simulink model "StewartPlatform"  (R2024a)
settings: Solver=ode8  StartTime=0.0  StopTime=inf  FixedStep=0.02  RelTol=1e-3  EnableMultiTasking=on
undefined symbols (not defined in the file or in its folder): Camera, Standard_Devices
libraries: pycoexlib x1, visionsinks x1, sldrtlib x1
settings Model: SimulationMode=external  ExtModeTrigDuration=2  Creator=Acrome  LastModifiedBy=burli
settings SolverCC: AlgebraicLoopSolver=TrustRegion
settings DataIOCC: ReturnWorkspaceOutputs=off
settings OptimizationCC: PassReuseOutputArgsAs=Individual arguments  MaxStackSize=64  EfficientTunableParamExpr=on
settings DebuggingCC: ParameterTunabilityLossMsg=error  UnconnectedInputMsg=warning  UnconnectedOutputMsg=warning  UnconnectedLineMsg=warning  ArithmeticOperatorsInVariantConditions=warning
settings HardwareCC: ProdBitPerInt=16  ProdBitPerPointer=16  ProdBitPerSizeT=16  ProdBitPerPtrDiffT=16  ProdLargestAtomicFloat=None  ProdWordSize=8  ProdHWDeviceType=Atmel->AVR
settings ModelReferenceCC: EnableRefExpFcnMdlSchedulingChecks=on
settings SFSimCC: SimUseLocalCustomCode=off  MATLABDynamicMemAlloc=off  CustomCodeUndefinedFunction=UseInterfaceOnly
settings RTWCC: Description=Embedded Coder  SystemTargetFile=ert.tlc  HardwareBoard=Arduino Mega 2560  TemplateMakefile=ert_default_tmf  GenerateReport=on  RTWUseLocalCustomCode=off  Toolchain=Arduino AVR  BuildConfiguration=Faster Runs  IncludeHyperlinkInReport=on  LaunchReport=on  GenerateTraceInfo=on  GenerateTraceReport=on  GenerateTraceReportSl=on  GenerateTraceReportSf=on  GenerateTraceReportEml=on  GPUComputeCapability=3.5
settings CodeAppCC: ForceParamTrailComments=on  IgnoreCustomStorageClasses=off  OperatorAnnotations=on  SimulinkDataObjDesc=on  SFDataObjDesc=on  InsertBlockDesc=on
settings ERTTargetCC: SupportContinuousTime=on  SupportVariableSizeSignals=on  ExtMode=on  ExtModeTransport=3  ExtModeStaticAlloc=on  ExtModeMexFile=ext_xcp  ExtModeMexArgs='127.0.0.1' 0 17725  ExtModeIntrfLevel=Level2 - Open

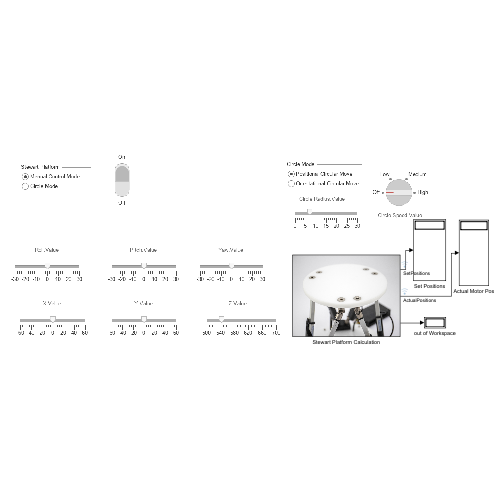
[thumbnail: Simulink's stored preview of the top-level diagram]
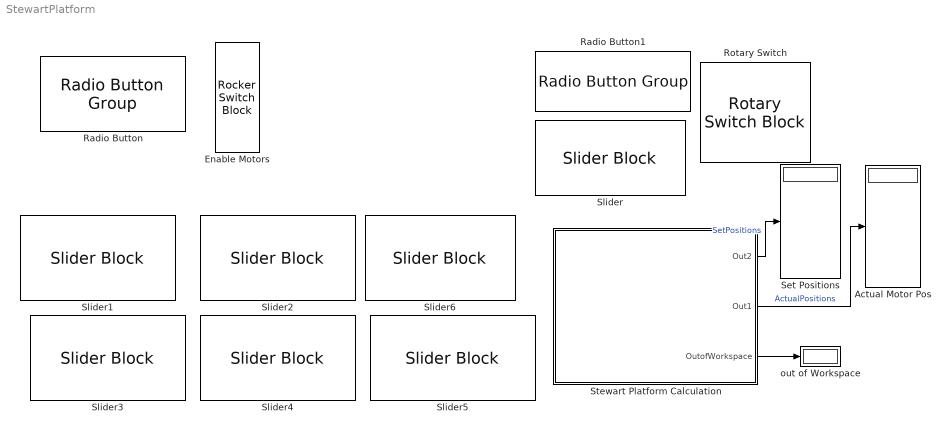
== system StewartPlatform ==
  Actual Motor Pos : Display
  Enable Motors : RockerSwitchBlock  LabelPosition=Hide
      settings: Values={{'Off', 'On'}, [0 1]}
  Radio Button : RadioButtonGroup  LabelPosition=Hide  SelectedLabel=Manual Control Mode  ButtonGroupName=Stewart Platform
      settings: Values={{'Manual Control Mode', 'Circle Mode'}, [0 1]}
  Radio Button1 : RadioButtonGroup  LabelPosition=Hide  SelectedLabel=Positional Circular Move  ButtonGroupName=Circle Mode
      settings: Values={{'Positional Circular Move', 'Orientational Circular Move'}, [0 1]}
  Rotary Switch : RotarySwitchBlock  LabelPosition=Bottom
      settings: Values={{'Off', 'Low', 'Medium', 'High'}, [0 2 3 4]}
  Set Positions : Display
  Slider : SliderBlock  ScaleMax=30
  Slider1 : SliderBlock  ScaleMin=-30  ScaleMax=30  TickInterval=10
  Slider2 : SliderBlock  ScaleMin=-30  ScaleMax=30  TickInterval=10
  Slider3 : SliderBlock  ScaleMin=-60  ScaleMax=60  TickInterval=20
  Slider4 : SliderBlock  ScaleMin=-60  ScaleMax=60  TickInterval=20
  Slider5 : SliderBlock  ScaleMin=500  ScaleMax=700
  Slider6 : SliderBlock  ScaleMin=-30  ScaleMax=30  TickInterval=10
  Stewart Platform Calculation : Subsystem
      mask Display: image('IMG_7112_1.jpg');
  out of Workspace : Display
  wires:
  Stewart Platform Calculation/2(Out1) -> Actual Motor Pos/1  "ActualPositions"
  Stewart Platform Calculation/1(Out2) -> Set Positions/1  "SetPositions"
  Stewart Platform Calculation/3(OutofWorkspace) -> out of Workspace/1

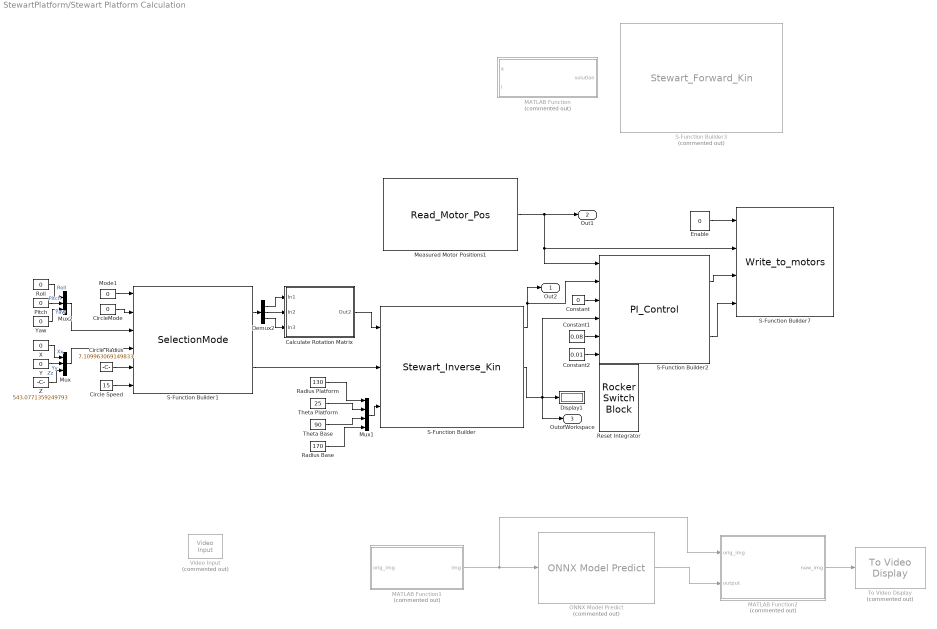
== system StewartPlatform/Stewart Platform Calculation ==
  " X" : Constant  Value=0
  Calculate Rotation Matrix : Subsystem
  Circle Radius : Constant  Value=7.109963069149833
  Circle Speed : Constant  Value=15
  CircleMode : Constant  Value=0  SampleTime=-1
  Constant : Constant  Value=0
  Constant1 : Constant  Value=0.08
  Constant2 : Constant  Value=0.01
  Demux2 : Demux  Outputs=3
  Display1 : Display
  Enable : Constant  Value=0
  MATLAB Function : MATLAB Function  Commented=on  TreatAsAtomicUnit=on
  MATLAB Function1 : MATLAB Function  Commented=on  TreatAsAtomicUnit=on
  MATLAB Function2 : MATLAB Function  Commented=on  TreatAsAtomicUnit=on
  Measured Motor Positions1 : S-Function  InitFcn=try, set_param(gcb,'FunctionName','Read_Motor_Pos'), end  FunctionName=Read_Motor_Pos  SFunctionModules=Read_Motor_Pos_wrapper.c  SFunctionDeploymentMode=off  EnableBusSupport=off  mask(S-Function Builder){}
      mask help: Simulink:masks:SFunctionBuilder_MD
      mask init:
      | val = [[.9  0.75 0.75 1 1 .9 .9 1]',[1 1 0.75 0.75 .9 .9 1 .9]'];try , sys = get_param(gcb,'SfunBuilderFcnName');if isempty(sys), sys = get_param(gcb,'FunctionName'); end,catch, sys = get_param(gcb,'FunctionName'); end
      settings: CopyFcn=set_param(gcbh,'LinkStatus','none')  PreSaveFcn=try, set_param(gcb,'FunctionName','Read_Motor_Pos'), end  OpenFcn=sfunctionwizard(gcbh)
      mask Display:
      | plot(val(:,1),val(:,2))
      | disp(sys)
      | port_label('output',1,'Mot_Pos')
  Mode1 : Constant  Value=0  SampleTime=-1
  Mux : Mux  Inputs=3
  Mux1 : Mux
  Mux2 : Mux  Inputs=3
  ONNX Model Predict : pycoexlib/ONNX Model Predict  Commented=on  ModelFile=C:\StewartProMatlab\SPro_Matlab_Mosfet v1_0_1\onnx_model_14.onnx  ExecutionProviders=CUDAExecutionProvider, CPUExecutionProvider  InputTable={ 'In1', 'float32', '[4 3 1 2]', 'inherit' }  OutputTable={ 'Out1', '', '' }  SampleTime=-1  InputDatatypes=float32  InputNumDims=inherit  InputPermutations=[4 3 1 2]  OutputPermutations=[]  PythonCoexecutionBlockType=ONNXModelBlock  VariableOutputMaxSizes=[]
  Pitch : Constant  Value=0  SampleTime=-1
  Radius Base : Constant  Value=170
  Radius Platform : Constant  Value=130
  Reset Integrator : RockerSwitchBlock  LabelPosition=Hide
      settings: Values={{'Off', 'On'}, [0 1]}
  Roll : Constant  Value=0  SampleTime=-1
  S-Function Builder : S-Function  InitFcn=try, set_param(gcb,'FunctionName','Stewart_Inverse_Kin'), end  FunctionName=Stewart_Inverse_Kin  SFunctionModules=Stewart_Inverse_Kin_wrapper  SFunctionDeploymentMode=off  EnableBusSupport=off  mask(S-Function Builder){}
      mask help: Simulink:masks:SFunctionBuilder_MD
      mask init: same as StewartPlatform/Stewart Platform Calculation/Measured Motor Positions1
      settings: CopyFcn=set_param(gcbh,'LinkStatus','none')  PreSaveFcn=try, set_param(gcb,'FunctionName','Stewart_Inverse_Kin'), end  OpenFcn=sfunctionwizard(gcbh)
      mask Display: plot(val(:,1),val(:,2)),disp(sys), port_label('input',1,'rotationmatrix'), port_label('input',2,'platform_pos'), port_label('input',3,'platform_parameters'), port_label('output',1,'Setpoints'), port_label('output',2,'outofWorkspace'), port_label('output',3,'y0')
  S-Function Builder1 : S-Function  InitFcn=try, set_param(gcb,'FunctionName','SelectionMode'), end  FunctionName=SelectionMode  SFunctionModules=SelectionMode_wrapper  SFunctionDeploymentMode=off  EnableBusSupport=off  mask(S-Function Builder){}
      mask help: Simulink:masks:SFunctionBuilder_MD
      mask init: same as StewartPlatform/Stewart Platform Calculation/Measured Motor Positions1
      settings: CopyFcn=set_param(gcbh,'LinkStatus','none')  PreSaveFcn=try, set_param(gcb,'FunctionName','SelectionMode'), end  OpenFcn=sfunctionwizard(gcbh)
      mask Display:
      | plot(val(:,1),val(:,2))
      | disp(sys)
      | port_label('input',1,'Mode')
      | port_label('input',2,'CircleMode')
      | port_label('input',3,'orientation_in')
      | port_label('input',4,'position_in')
      | port_label('input',5,'Radius')
      | port_label('input',6,'Speed')
      | port_label('output',1,'orientation_out')
      | port_label('output',2,'position_out')
  S-Function Builder2 : S-Function  InitFcn=try, set_param(gcb,'FunctionName','PI_Control'), end  FunctionName=PI_Control  SFunctionModules=PI_Control_wrapper  SFunctionDeploymentMode=off  EnableBusSupport=off  mask(S-Function Builder){}
      mask help: Simulink:masks:SFunctionBuilder_MD
      mask init: same as StewartPlatform/Stewart Platform Calculation/Measured Motor Positions1
      settings: CopyFcn=set_param(gcbh,'LinkStatus','none')  PreSaveFcn=try, set_param(gcb,'FunctionName','PI_Control'), end  OpenFcn=sfunctionwizard(gcbh)
      mask Display: plot(val(:,1),val(:,2)),disp(sys), port_label('input',1,'ActualPos'), port_label('input',2,'SetPos'), port_label('input',3,'ResetIntegrator'), port_label('input',4,'inWorkSpace'), port_label('input',5,'P'), port_label('input',6,'I'), port_label('output',1,'PWMOut'), port_label('output',2,'Directions')
  S-Function Builder3 : S-Function  Commented=on  FunctionName=Stewart_Forward_Kin  SFunctionModules=Stewart_Forward_Kin_wrapper.c  SFunctionDeploymentMode=off  EnableBusSupport=off  mask(S-Function Builder){}
      mask help: Simulink:masks:SFunctionBuilder_MD
      mask init: same as StewartPlatform/Stewart Platform Calculation/Measured Motor Positions1
      settings: CopyFcn=set_param(gcbh,'LinkStatus','none')  OpenFcn=sfunctionwizard(gcbh)
      mask Display:
      | plot(val(:,1),val(:,2))
      | disp(sys)
      | port_label('input',1,'actual_lengths')
      | port_label('input',2,'platform_parameters')
      | port_label('output',1,'actual_pos')
  S-Function Builder7 : S-Function  InitFcn=try, set_param(gcb,'FunctionName','Write_to_motors'), end  FunctionName=Write_to_motors  SFunctionModules=Write_to_motors_wrapper  SFunctionDeploymentMode=off  EnableBusSupport=off  mask(S-Function Builder){}
      mask help: Simulink:masks:SFunctionBuilder_MD
      mask init: same as StewartPlatform/Stewart Platform Calculation/Measured Motor Positions1
      settings: CopyFcn=set_param(gcbh,'LinkStatus','none')  PreSaveFcn=try, set_param(gcb,'FunctionName','Write_to_motors'), end  OpenFcn=sfunctionwizard(gcbh)
      mask Display: plot(val(:,1),val(:,2)),disp(sys),port_label('input',1,'EnabledMotors'),port_label('input',2,'MotorPos'),port_label('input',3,'PWMin'),port_label('input',4,'Direction')
  Theta Base : Constant  Value=90
  Theta Platform : Constant  Value=25
  To Video Display : visionsinks/To Video Display  Commented=on  windowSizeMode=Normal  openAtMdlStart=on  fullScreen=off  videoWindowX=536805376  videoWindowY=536805376  saveWindowSize=off  videoWindowWidth=2147483647  videoWindowHeight=2147483647  inputColorFormat=RGB  inputType=Obsolete  imagePorts=One multidimensional signal  OutputDevice=On-screen video monitor  dataOrg=Column-major  isWindowOpen=off
  Video Input : sldrtlib/Video Input  Commented=on  SampleTime=0.1  MaxMissedTicks=10  ShowMissedTicks=off  YieldWhenWaiting=off  DrvName=Standard_Devices/Camera  DrvAddress=1  DrvOptions=[320 240 1]  Channels=[1 2 3]  RoiOriginSource=1  RoiOrigin=[1 1]  RoiDimensions=[320 240]  ShowReady=off  ShowError=off  ShowTimestamp=off
      settings: AttributesFormatString=Camera [1]
  Y : Constant  Value=0
  Yaw : Constant  Value=0  SampleTime=-1
  Z : Constant  Value=543.0771359249793
  Out2 : Outport  VectorParamsAs1DForOutWhenUnconnected=off
  Out1 : Outport  Port=2  VectorParamsAs1DForOutWhenUnconnected=off
  OutofWorkspace : Outport  Port=3  VectorParamsAs1DForOutWhenUnconnected=off
  wires:
  Z/1 -> Mux/3  "Zz"
  Y/1 -> Mux/2  "Yy"
  " X"/1 -> Mux/1  "Xx"
  Mode1/1 -> S-Function Builder1/1
  CircleMode/1 -> S-Function Builder1/2
  Mux2/1 -> S-Function Builder1/3
  Yaw/1 -> Mux2/3  "Yaw"
  Pitch/1 -> Mux2/2  "Pitch"
  Roll/1 -> Mux2/1  "Roll"
  Circle Radius/1 -> S-Function Builder1/5
  Circle Speed/1 -> S-Function Builder1/6
  Mux/1 -> S-Function Builder1/4
  Demux2/2 -> Calculate Rotation Matrix/2(In2)
  Demux2/1 -> Calculate Rotation Matrix/1(In1)
  S-Function Builder1/1 -> Demux2/1
  Demux2/3 -> Calculate Rotation Matrix/3(In3)
  S-Function Builder1/2 -> S-Function Builder/2
  Theta Platform/1 -> Mux1/2
  Calculate Rotation Matrix/1(Out2) -> S-Function Builder/1
  Mux1/1 -> S-Function Builder/3
  Radius Platform/1 -> Mux1/1
  Radius Base/1 -> Mux1/4
  Theta Base/1 -> Mux1/3
  Enable/1 -> S-Function Builder7/1
  Constant/1 -> S-Function Builder2/3
  S-Function Builder/2 -> Display1/1, S-Function Builder2/4, OutofWorkspace/1
  Constant1/1 -> S-Function Builder2/5
  Constant2/1 -> S-Function Builder2/6
  S-Function Builder2/1 -> S-Function Builder7/3
  S-Function Builder2/2 -> S-Function Builder7/4
  S-Function Builder/1 -> S-Function Builder2/2, Out2/1
  Measured Motor Positions1/1 -> S-Function Builder7/2, S-Function Builder2/1, Out1/1
  MATLAB Function2/1(new_img) -> To Video Display/1
  MATLAB Function1/1(img) -> MATLAB Function2/1(orig_img), ONNX Model Predict/1
  ONNX Model Predict/1 -> MATLAB Function2/2(output)

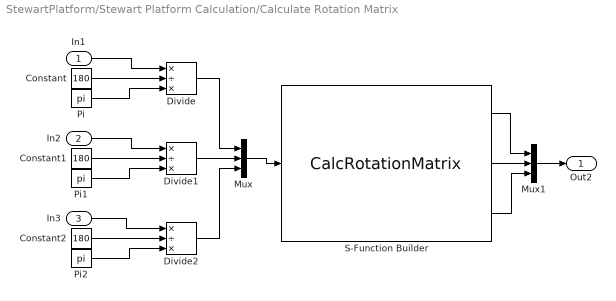
== system StewartPlatform/Stewart Platform Calculation/Calculate Rotation Matrix ==
  In1 : Inport
  In2 : Inport  Port=2
  In3 : Inport  Port=3
  Constant : Constant  Value=180  SampleTime=-1
  Constant1 : Constant  Value=180  SampleTime=-1
  Constant2 : Constant  Value=180  SampleTime=-1
  Divide : Product  Inputs=*/*
  Divide1 : Product  Inputs=*/*
  Divide2 : Product  Inputs=*/*
  Mux : Mux  Inputs=3
  Mux1 : Mux  Inputs=3
  Pi : Constant  Value=pi  SampleTime=-1
  Pi1 : Constant  Value=pi  SampleTime=-1
  Pi2 : Constant  Value=pi  SampleTime=-1
  S-Function Builder : S-Function  InitFcn=try, set_param(gcb,'FunctionName','CalcRotationMatrix'), end  FunctionName=CalcRotationMatrix  SFunctionModules=CalcRotationMatrix_wrapper  SFunctionDeploymentMode=off  EnableBusSupport=off  mask(S-Function Builder){}
      mask help: Simulink:masks:SFunctionBuilder_MD
      mask init: same as StewartPlatform/Stewart Platform Calculation/Measured Motor Positions1
      settings: CopyFcn=set_param(gcbh,'LinkStatus','none')  PreSaveFcn=try, set_param(gcb,'FunctionName','CalcRotationMatrix'), end  OpenFcn=sfunctionwizard(gcbh)
      mask Display:
      | plot(val(:,1),val(:,2))
      | disp(sys)
      | port_label('input',1,'angles')
      | port_label('output',1,'out')
      | port_label('output',2,'out1')
      | port_label('output',3,'out2')
  Out2 : Outport  VectorParamsAs1DForOutWhenUnconnected=off
  wires:
  In3/1 -> Divide2/1
  In2/1 -> Divide1/1
  Pi/1 -> Divide/3
  Divide1/1 -> Mux/2
  Pi2/1 -> Divide2/3
  Pi1/1 -> Divide1/3
  Constant/1 -> Divide/2
  Constant2/1 -> Divide2/2
  Divide2/1 -> Mux/3
  Constant1/1 -> Divide1/2
  Divide/1 -> Mux/1
  Mux/1 -> S-Function Builder/1
  In1/1 -> Divide/1
  S-Function Builder/1 -> Mux1/1
  S-Function Builder/2 -> Mux1/2
  S-Function Builder/3 -> Mux1/3
  Mux1/1 -> Out2/1

== matlab function StewartPlatform/Stewart Platform Calculation/MATLAB Function1 ==
  data: orig_img input; img output
function img = preProcess(orig_img)
% 240,320,3
img=double(orig_img)/255.0;

== matlab function StewartPlatform/Stewart Platform Calculation/MATLAB Function ==
  data: a input; solution output size=6; l input

function solution = stewart_forward(a,l)

    num=0;
    tolf = 1e-6;
    tola = 1e-6;
    maxiter = 1e3;
    platform_parameters=[130,25,90,170]; %p r, p theta, b theta, b r
    top_offset = [0;0;62];
    base_offset = [0;0;57];

    while num<maxiter
        % convert deg to rad
        gamma=a(4)*pi/180;
        beta=a(5)*pi/180;
        alpha=a(6)*pi/180;
    
        sumf=0; % to sum fi(a)
        n=0;m=0;
    
        % define func, B for i 1-6
        func = zeros(1,6);
        A = zeros(6,6);
        B = zeros(6,1);
    
        % compute rotation matrix
        R = [cos(gamma)*cos(beta), cos(gamma)*sin(beta)*sin(alpha)-sin(gamma)*cos(alpha), cos(gamma)*sin(beta)*cos(alpha)+sin(gamma)*sin(alpha);
            sin(gamma)*cos(beta), sin(gamma)*sin(beta)*sin(alpha)+cos(gamma)*cos(alpha), sin(gamma)*sin(beta)*cos(alpha)-cos(gamma)*sin(alpha);
            -sin(beta), cos(beta)*sin(alpha), cos(beta)*cos(alpha)];
    
        % adjust x, y, z
        x=a(1);
        y=a(2);
        z=a(3);
        a2 = R*top_offset+base_offset;
        x=x-a2(1);
        y=y-a2(2);
        z=z-a2(3);
    
        for i = 1:6
            b=mod(i,2);
            if b==1
                n=(60*i)-(platform_parameters(2)/2);
                m=(60*i)-(platform_parameters(3)/2); 
            else
                n=n+platform_parameters(2);
                m=m+platform_parameters(3);
            end
            
            
            % calculate xb = db - bb
            bB=[platform_parameters(4)*cos((m/180.0)*pi);
                platform_parameters(4)*sin((m/180.0)*pi);
                0];
            xB=[x-bB(1),y-bB(2),z-bB(3)];
    
            % calculate pb = R*pp
            pP=[platform_parameters(1)*cos((n/180.0)*pi);
                platform_parameters(1)*sin((n/180.0)*pi);
                0];
            pB = R*pP;
    
    
            % compute fi(a)
            func(i) = (xB(1)+pB(1))^2 + (xB(2)+pB(2))^2 + (xB(3)+pB(3))^2 - l(i)^2;
            sumf = sumf + abs(func(i)); % add to sum of fi(a)
            B(i) = -func(i);
    
            % compute A partial derivatives
            A(i,1)=2*(xB(1)+pB(1));
            A(i,2)=2*(xB(2)+pB(2));
            A(i,3)=2*(xB(3)+pB(3));
            A(i,4)=2*(-xB(1)*pB(2)+xB(2)*pB(1));
            A(i,5)=2*(pB(3)*(-xB(1)*cos(gamma)+xB(2)*sin(gamma))-xB(3)*(pP(1)*cos(beta)+pP(2)*sin(beta)*sin(alpha)));
            A(i,6)=2*pP(2)*(xB(1)*R(1,3)+xB(2)*R(2,3)+xB(3)*R(3,3));
        
        end
    
        if sumf < tolf
            a([4 6]) = a([6 4]);
            solution = a;
            return
        end
    
        % LU decomp step, solve for delta a (j): A*deltaa=B
        deltaa = A\B;
        deltaa(4:6)=deltaa(4:6)*180/pi; % convert back to deg
        if sum(abs(deltaa)) < tola
            a([4 6]) = a([6 4]);
            solution = a;
            return
        end
    
        if num>maxiter
            a([4 6]) = a([6 4]);
            solution = a;
            return
        end
    
        num=num+1;
        a=a+ deltaa;
    end
    solution=a;
    % disp(solution);
end

== matlab function StewartPlatform/Stewart Platform Calculation/MATLAB Function2 ==
  data: orig_img input; new_img output; output input
function new_img = postProcess(orig_img,output)

    orig_img = permute(orig_img,[3,1,2]);
    c = orig_img(1,:,:)+output;
    orig_img(1,:,:) = c./max(c,[],'all');

    orig_img = permute(orig_img,[2,3,1]);
    new_img = uint8(round(orig_img*255));
